simulink model "ChirpTest"  (R2019b)
settings: Solver=VariableStepAuto  StartTime=0.0  StopTime=PWM.Time(end)  MaxStep=1/(PWM_Resolution*PWM_Frequency)  RelTol=1e-3
PreLoadFcn:
  | modelDir = fileparts(get_param(bdroot, 'FileName'));
  | addpath(fullfile(modelDir,'../Parameters'));
  | addpath(fullfile(modelDir,'subsystems'));
  | addpath(fullfile(modelDir,'../DesignExploration/functions')); % for PWM_Generator
  | 
  | Parameters_Model
  | Parameters_Simulation
  | Parameters_Test_Chirp
InitFcn:
  | Parameters_Model
  | Parameters_Simulation
  | Parameters_Test_Chirp
undefined symbols (not defined in the file): chirp_duty_cycle, chirp_t_end
libraries: simulink x4
settings Model: Creator=Thomas  LastModifiedBy=thomas.jespersen
settings DataIOCC: ReturnWorkspaceOutputs=off
settings DebuggingCC: ArithmeticOperatorsInVariantConditions=warning
settings SFSimCC: SimUseLocalCustomCode=off  CustomCodeUndefinedFunction=UseInterfaceOnly
settings RTWCC: RTWUseLocalCustomCode=off

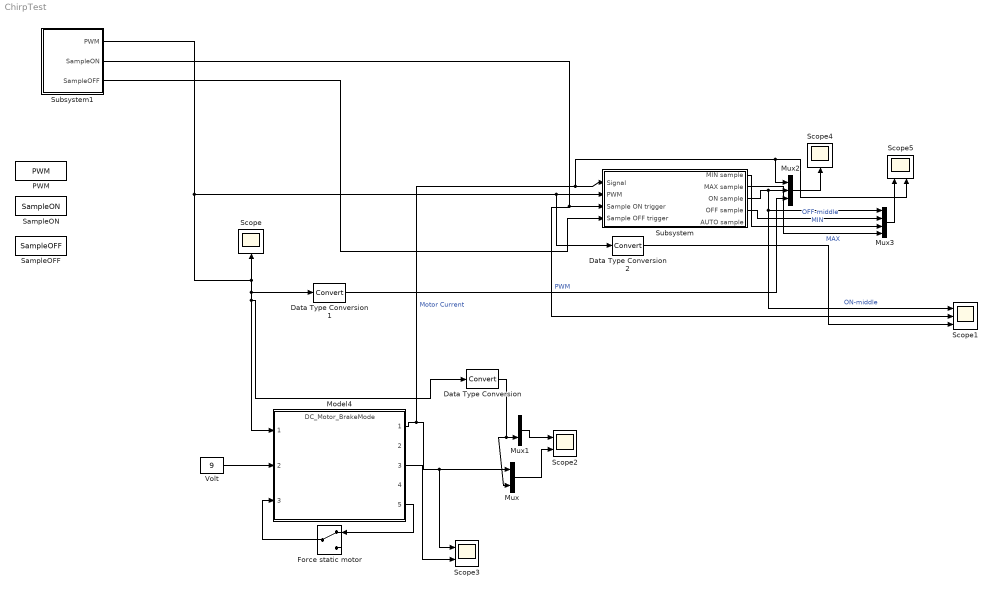
== system ChirpTest ==
  Data Type Conversion : DataTypeConversion  RndMeth=Round
  Data Type Conversion1 : DataTypeConversion  RndMeth=Round
  Data Type Conversion2 : DataTypeConversion  RndMeth=Round
  Force static motor : ManualSwitch
  Model4 : ModelReference  ModelNameDialog=DC_Motor_BrakeMode  SimulationMode=Normal  ModelReferenceVersion=1.43
  Mux : Mux  Inputs=2
  Mux1 : Mux  Inputs=2
  Mux2 : Mux  Inputs=3
  Mux3 : Mux
  PWM : FromWorkspace  VariableName=PWM  SampleTime=0  Interpolate=off  OutputAfterFinalValue=Holding final value
  SampleOFF : FromWorkspace  VariableName=SampleOFF  SampleTime=0  Interpolate=off  OutputAfterFinalValue=Holding final value
  SampleON : FromWorkspace  VariableName=SampleON  SampleTime=0  Interpolate=off  OutputAfterFinalValue=Holding final value
  Scope : Scope
  Scope1 : Scope  NumInputPorts=3
  Scope2 : Scope  NumInputPorts=2
  Scope3 : Scope  NumInputPorts=2
  Scope4 : Scope
  Scope5 : Scope  NumInputPorts=2
  Subsystem : Subsystem
  Subsystem1 : Subsystem
  Volt : Constant  Value=9
  wires:
  Volt/1 -> Model4/2
  Model4/1 -> Scope5/2, Mux2/1, Subsystem/1(Signal), Scope3/1, Mux/1  "Motor Current"
  Mux/1 -> Scope2/2
  Mux1/1 -> Scope2/1
  Data Type Conversion/1 -> Mux/2, Mux1/2
  Model4/3 -> Scope3/2
  Mux2/1 -> Scope4/1
  Subsystem/3(ON sample) -> Scope1/1, Mux3/1, Mux2/2  "ON-middle"
  Mux3/1 -> Scope5/1
  Subsystem/4(OFF sample) -> Mux3/2  "OFF-middle"
  Subsystem/1(MIN sample) -> Mux3/3  "MIN"
  Subsystem/2(MAX sample) -> Mux3/4  "MAX"
  Data Type Conversion2/1 -> Scope1/3
  Force static motor/1 -> Model4/3
  Subsystem1/1(PWM) -> Data Type Conversion1/1, Model4/1, Data Type Conversion/1, Scope/1, Data Type Conversion2/1, Subsystem/2(PWM)
  Subsystem1/3(SampleOFF) -> Subsystem/4(Sample OFF trigger)
  Subsystem1/2(SampleON) -> Scope1/2, Subsystem/3(Sample ON trigger)
  Data Type Conversion1/1 -> Mux2/3  "PWM"
  Model4/5 -> Force static motor/1

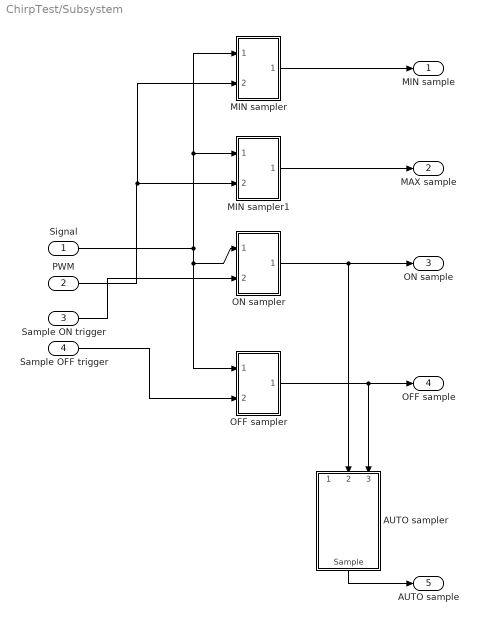
== system ChirpTest/Subsystem ==
  Signal : Inport
  PWM : Inport  Port=2
  Sample ON trigger : Inport  Port=3
  Sample OFF trigger : Inport  Port=4
  AUTO sampler : Subsystem
  MIN sampler : Subsystem
  MIN sampler1 : Subsystem
  OFF sampler : Subsystem
  ON sampler : Subsystem
  MIN sample : Outport  VectorParamsAs1DForOutWhenUnconnected=off
  MAX sample : Outport  Port=2  VectorParamsAs1DForOutWhenUnconnected=off
  ON sample : Outport  Port=3  VectorParamsAs1DForOutWhenUnconnected=off
  OFF sample : Outport  Port=4  VectorParamsAs1DForOutWhenUnconnected=off
  AUTO sample : Outport  Port=5  VectorParamsAs1DForOutWhenUnconnected=off
  wires:
  Signal/1 -> OFF sampler/1(Signal), ON sampler/1(Signal), MIN sampler1/1(Signal), MIN sampler/1(Signal)
  ON sampler/1(Sample) -> AUTO sampler/2(ON sample), ON sample/1
  OFF sampler/1(Sample) -> AUTO sampler/3(OFF sample), OFF sample/1
  AUTO sampler/1(Sample) -> AUTO sample/1
  MIN sampler1/1(Sample) -> MAX sample/1
  MIN sampler/1(Sample) -> MIN sample/1
  PWM/1 -> MIN sampler/2(PWM), MIN sampler1/2(PWM)
  Sample OFF trigger/1 -> OFF sampler/2(Trigger)
  Sample ON trigger/1 -> ON sampler/2(Trigger)

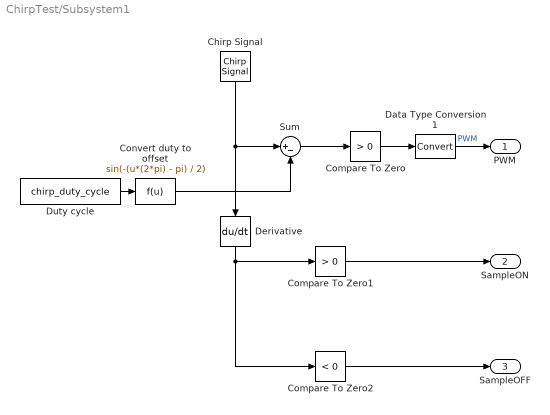
== system ChirpTest/Subsystem1 ==
  Chirp Signal : simulink/Sources/Chirp Signal  f1=chirp_freq_start  T=chirp_t_end  f2=chirp_freq_end
  Compare To Zero : simulink/Logic and Bit Operations/Compare To Zero  relop=>  OutDataTypeStr=boolean
  Compare To Zero1 : simulink/Logic and Bit Operations/Compare To Zero  relop=>  OutDataTypeStr=boolean  ZeroCross=off
  Compare To Zero2 : simulink/Logic and Bit Operations/Compare To Zero  relop=<  OutDataTypeStr=boolean  ZeroCross=off
  Convert duty to offset : Fcn  Expr=sin(-(u*(2*pi) - pi) / 2)
  Data Type Conversion1 : DataTypeConversion  RndMeth=Round
  Derivative : Derivative
  Duty cycle : Constant  Value=chirp_duty_cycle
  Sum : Sum  Inputs=|+-
  PWM : Outport  OutDataTypeStr=int8  VectorParamsAs1DForOutWhenUnconnected=off
  SampleON : Outport  Port=2  VectorParamsAs1DForOutWhenUnconnected=off
  SampleOFF : Outport  Port=3  VectorParamsAs1DForOutWhenUnconnected=off
  wires:
  Duty cycle/1 -> Convert duty to offset/1
  Sum/1 -> Compare To Zero/1
  Convert duty to offset/1 -> Sum/2
  Compare To Zero/1 -> Data Type Conversion1/1
  Compare To Zero1/1 -> SampleON/1
  Chirp Signal/1 -> Derivative/1, Sum/1
  Compare To Zero2/1 -> SampleOFF/1
  Derivative/1 -> Compare To Zero2/1, Compare To Zero1/1
  Data Type Conversion1/1 -> PWM/1  "PWM"

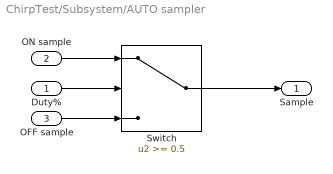
== system ChirpTest/Subsystem/AUTO sampler ==
  Duty% : Inport  OutDataTypeStr=double
  ON sample : Inport  Port=2
  OFF sample : Inport  Port=3
  Switch : Switch  Threshold=0.5
  Sample : Outport  VectorParamsAs1DForOutWhenUnconnected=off
  wires:
  Duty%/1 -> Switch/2
  ON sample/1 -> Switch/1
  OFF sample/1 -> Switch/3
  Switch/1 -> Sample/1

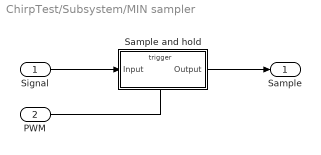
== system ChirpTest/Subsystem/MIN sampler ==
  Signal : Inport
  PWM : Inport  Port=2
  Sample and hold : Subsystem
  Sample : Outport  VectorParamsAs1DForOutWhenUnconnected=off
  wires:
  Signal/1 -> Sample and hold/1(Input)
  Sample and hold/1(Output) -> Sample/1
  PWM/1 -> Sample and hold/Trigger

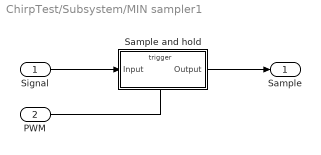
== system ChirpTest/Subsystem/MIN sampler1 ==
  Signal : Inport
  PWM : Inport  Port=2
  Sample and hold : Subsystem
  Sample : Outport  VectorParamsAs1DForOutWhenUnconnected=off
  wires:
  Signal/1 -> Sample and hold/1(Input)
  Sample and hold/1(Output) -> Sample/1
  PWM/1 -> Sample and hold/Trigger

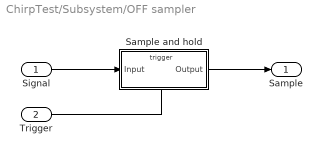
== system ChirpTest/Subsystem/OFF sampler ==
  Signal : Inport
  Trigger : Inport  Port=2
  Sample and hold : Subsystem
  Sample : Outport  VectorParamsAs1DForOutWhenUnconnected=off
  wires:
  Signal/1 -> Sample and hold/1(Input)
  Sample and hold/1(Output) -> Sample/1
  Trigger/1 -> Sample and hold/Trigger

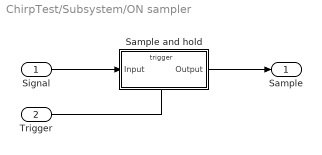
== system ChirpTest/Subsystem/ON sampler ==
  Signal : Inport
  Trigger : Inport  Port=2
  Sample and hold : Subsystem
  Sample : Outport  VectorParamsAs1DForOutWhenUnconnected=off
  wires:
  Signal/1 -> Sample and hold/1(Input)
  Sample and hold/1(Output) -> Sample/1
  Trigger/1 -> Sample and hold/Trigger

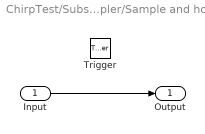
== system ChirpTest/Subsystem/MIN sampler/Sample and hold ==
  Input : Inport
  Trigger : TriggerPort  VariantControl=Variant  PortDimensions=1
  Output : Outport  VectorParamsAs1DForOutWhenUnconnected=off
  wires:
  Input/1 -> Output/1

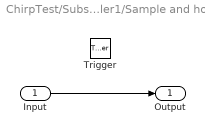
== system ChirpTest/Subsystem/MIN sampler1/Sample and hold ==
  Input : Inport
  Trigger : TriggerPort  TriggerType=falling  VariantControl=Variant  PortDimensions=1
  Output : Outport  VectorParamsAs1DForOutWhenUnconnected=off
  wires:
  Input/1 -> Output/1

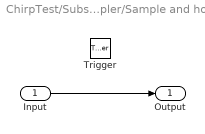
== system ChirpTest/Subsystem/OFF sampler/Sample and hold ==
  Input : Inport
  Trigger : TriggerPort  TriggerType=falling  VariantControl=Variant  PortDimensions=1
  Output : Outport  VectorParamsAs1DForOutWhenUnconnected=off
  wires:
  Input/1 -> Output/1

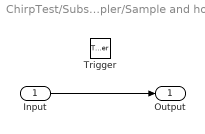
== system ChirpTest/Subsystem/ON sampler/Sample and hold ==
  Input : Inport
  Trigger : TriggerPort  TriggerType=falling  VariantControl=Variant  PortDimensions=1
  Output : Outport  VectorParamsAs1DForOutWhenUnconnected=off
  wires:
  Input/1 -> Output/1
